simulink model "FA_18_MPC_Multiple_Actuator"  (R2018a)
settings: Solver=ode45  StartTime=0.0  StopTime=150  RelTol=1e-3
libraries: simulink_extras x3, mpclib x1
settings Model: Creator=User  LastModifiedBy=User
settings CodeAppCC: StateflowObjectComments=on

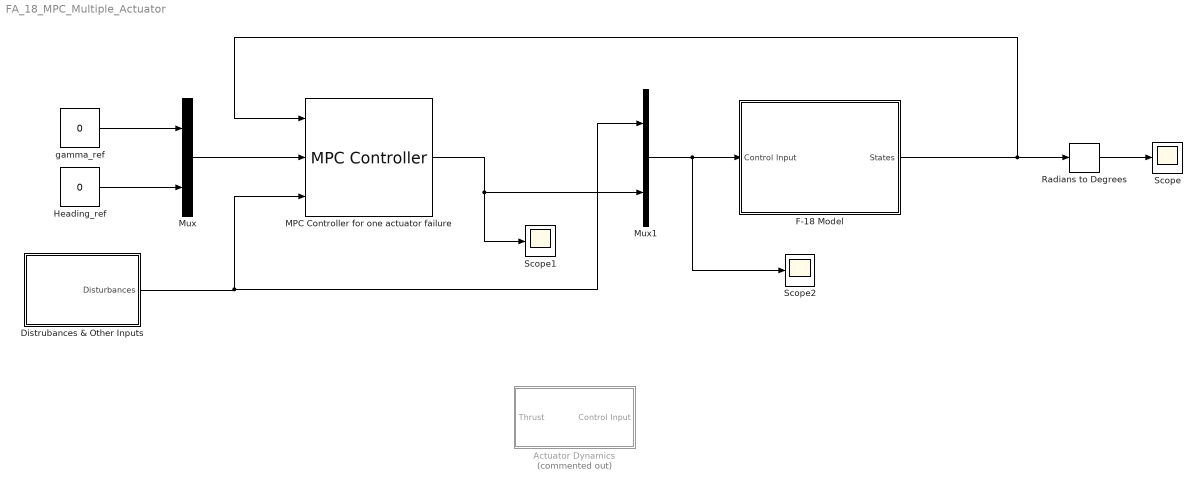
== system FA_18_MPC_Multiple_Actuator ==
  Actuator Dynamics : Subsystem  Commented=on
  Distrubances & Other Inputs : Subsystem
  F-18 Model : Subsystem
  Heading_ref : Constant  Value=0
  MPC Controller for one actuator failure : mpclib/MPC Controller  SCDEnableBlockLinearizationSpecification=on  mpcobj=mpc1  is_multiple=0  enable_value=0  return_u0=off  updateMPCinCallerWorkspace=on  ref_from_ws=off  ref_signal_name=[]  ref_preview=off  md_from_ws=off  md_signal_name=[]  md_preview=off  from_project=off  project_file=MPCtask.mat  md_inport=on  mv_inport=off  cost_outport=off  return_sequence=off  return_qpstatus=off  return_state=off  state_inport=off  lims_inport=off  cc_inport=off  ywt_inport=off  is_designfromscratch=0  uwt_inport=off  duwt_inport=off  rhoeps_inport=off  uref_inport=off  n_ts=0.1  n_p=10  n_mv=2  n_md=2  n_ud=0  n_mo=2  n_uo=0  BlockDataType=double  SampleTimeInherited=off  switch_inport=off
  Mux : Mux  Inputs=2
  Mux1 : Mux  Inputs=2
  Radians to Degrees : simulink_extras/Transformations/Radians to Degrees
  Scope : Scope
  Scope1 : Scope
  Scope2 : Scope
  gamma_ref : Constant  Value=0
  wires:
  F-18 Model/1(States) -> MPC Controller for one actuator failure/1, Radians to Degrees/1
  Distrubances & Other Inputs/1(Disturbances) -> Mux1/1, MPC Controller for one actuator failure/3
  MPC Controller for one actuator failure/1 -> Scope1/1, Mux1/2
  Mux1/1 -> Scope2/1, F-18 Model/1(Control Input)
  Radians to Degrees/1 -> Scope/1
  gamma_ref/1 -> Mux/1
  Mux/1 -> MPC Controller for one actuator failure/2
  Heading_ref/1 -> Mux/2

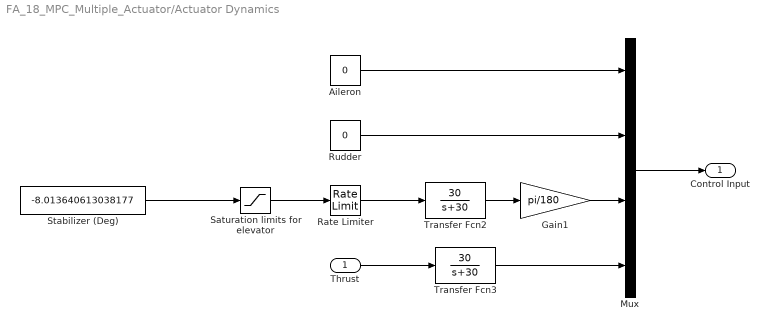
== system FA_18_MPC_Multiple_Actuator/Actuator Dynamics ==
  Thrust : Inport
  Aileron : Constant  Value=0
  Gain1 : Gain  Gain=pi/180
  Mux : Mux
  Rate Limiter : RateLimiter  RisingSlewLimit=40  FallingSlewLimit=-40  SampleTimeMode=inherited
  Rudder : Constant  Value=0
  Saturation limits for elevator : Saturate  UpperLimit=10.5  LowerLimit=-24
  Stabilizer (Deg) : Constant  Value=-8.013640613038177
  Transfer Fcn2 : TransferFcn  Numerator=[30]  Denominator=[1 30]
  Transfer Fcn3 : TransferFcn  Numerator=[30]  Denominator=[1 30]
  Control Input : Outport
  wires:
  Mux/1 -> Control Input/1
  Aileron/1 -> Mux/1
  Transfer Fcn3/1 -> Mux/4
  Rudder/1 -> Mux/2
  Thrust/1 -> Transfer Fcn3/1
  Saturation limits for elevator/1 -> Rate Limiter/1
  Rate Limiter/1 -> Transfer Fcn2/1
  Stabilizer (Deg)/1 -> Saturation limits for elevator/1
  Gain1/1 -> Mux/3
  Transfer Fcn2/1 -> Gain1/1

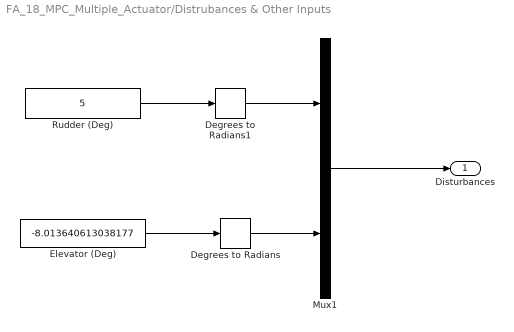
== system FA_18_MPC_Multiple_Actuator/Distrubances & Other Inputs ==
  Degrees to Radians : simulink_extras/Transformations/Degrees to Radians
  Degrees to Radians1 : simulink_extras/Transformations/Degrees to Radians
  Elevator (Deg) : Constant  Value=-8.013640613038177
  Mux1 : Mux  Inputs=2
  Rudder (Deg) : Constant  Value=5
  Disturbances : Outport
  wires:
  Mux1/1 -> Disturbances/1
  Degrees to Radians/1 -> Mux1/2
  Elevator (Deg)/1 -> Degrees to Radians/1
  Rudder (Deg)/1 -> Degrees to Radians1/1
  Degrees to Radians1/1 -> Mux1/1

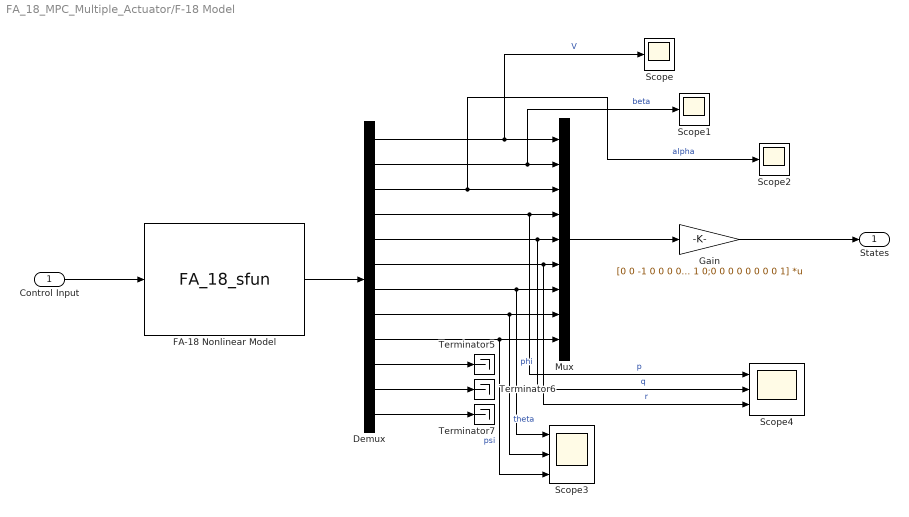
== system FA_18_MPC_Multiple_Actuator/F-18 Model ==
  Control Input : Inport
  Demux : Demux  Outputs=12
  FA-18 Nonlinear Model : S-Function  FunctionName=FA_18_sfun  SFunctionDeploymentMode=off  EnableBusSupport=off
  Gain : Gain  Gain=[0 0 -1 0 0 0 0 1 0;0 0 0 0 0 0 0 0 1]  Multiplication=Matrix(K*u)
  Mux : Mux  Inputs=9
  Scope : Scope
  Scope1 : Scope
  Scope2 : Scope
  Scope3 : Scope  NumInputPorts=3
  Scope4 : Scope  NumInputPorts=3
  Terminator5 : Terminator
  Terminator6 : Terminator
  Terminator7 : Terminator
  States : Outport
  wires:
  Control Input/1 -> FA-18 Nonlinear Model/1
  FA-18 Nonlinear Model/1 -> Demux/1
  Demux/1 -> Scope/1, Mux/1  "V"
  Demux/5 -> Scope4/2, Mux/5  "q"
  Demux/8 -> Scope3/2, Mux/8  "theta"
  Demux/2 -> Scope1/1, Mux/2  "beta"
  Demux/4 -> Scope4/1, Mux/4  "p"
  Demux/6 -> Scope4/3, Mux/6  "r"
  Demux/7 -> Scope3/1, Mux/7  "phi"
  Demux/10 -> Terminator5/1
  Demux/11 -> Terminator6/1
  Demux/12 -> Terminator7/1
  Mux/1 -> Gain/1
  Demux/9 -> Scope3/3, Mux/9  "psi"
  Demux/3 -> Scope2/1, Mux/3  "alpha"
  Gain/1 -> States/1
